simulink subsystem "subsys_Full_Model_NL"  (R2021a)
settings: Solver=VariableStepAuto  StartTime=0.0  StopTime=10.0  RelTol=1e-3
values from neighbouring files (symbols this model uses):
  g = 9.81    [Constante_NL.m]
  LL = .115    (= 0.115)    [Constante_NL.m]
  mP = masseP    (= 0.425)    [Constante_NL.m]
  RR = 3.6    [Constante_NL.m]
  sig = 1    [Constante_NL.m]
  XA = +rABC    (= 0.0952)    [Constante_NL.m]
  XB = -rABC*sind(30)    [Constante_NL.m]
  XC = -rABC*sind(30)    [Constante_NL.m]
  XD = +rDEF*sind(30)    [Constante_NL.m]
  XE = -rDEF    (= -0.08)    [Constante_NL.m]
  XF = +rDEF*sind(30)    [Constante_NL.m]
  YA = 0.0    (= 0)    [Constante_NL.m]
  YB = +rABC*cosd(30)    [Constante_NL.m]
  YC = -rABC*cosd(30)    [Constante_NL.m]
  YD = +rDEF*cosd(30)    [Constante_NL.m]
  YE = 0.0    (= 0)    [Constante_NL.m]
  YF = -rDEF*cosd(30)    [Constante_NL.m]
undefined symbols (not defined in the file or in its folder): Jx, mS
settings Model: Creator=antho  LastModifiedBy=antho

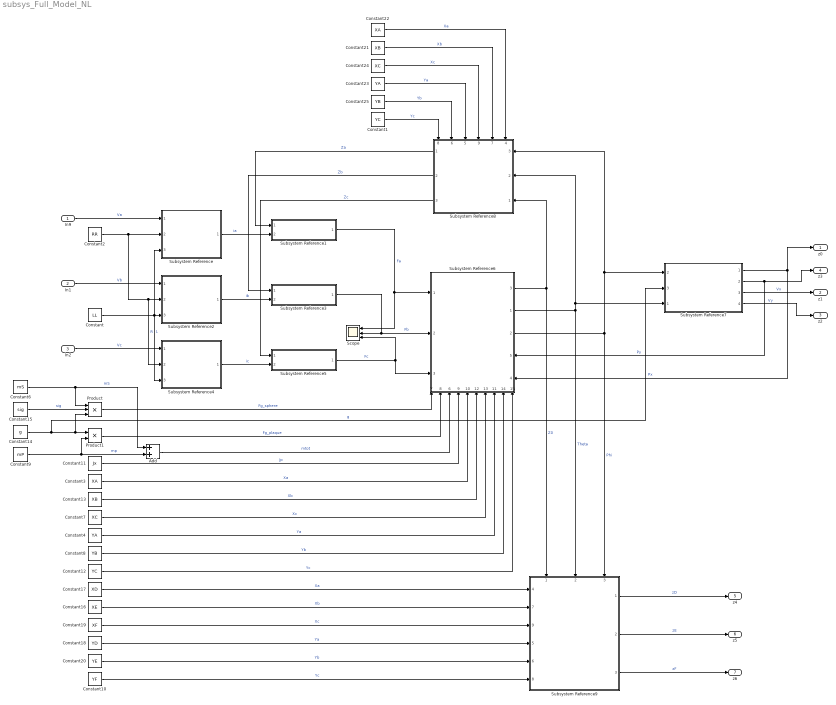
== system subsys_Full_Model_NL ==
  In9 : Inport
  In1 : Inport  Port=2
  In2 : Inport  Port=3
  Add : Sum
  Constant : Constant  Value=LL
  Constant1 : Constant  Value=YC
  Constant10 : Constant  Value=YF
  Constant11 : Constant  Value=Jx
  Constant12 : Constant  Value=YC
  Constant13 : Constant  Value=XB
  Constant14 : Constant  Value=g
  Constant15 : Constant  Value=sig
  Constant16 : Constant  Value=XE
  Constant17 : Constant  Value=XD
  Constant18 : Constant  Value=YD
  Constant19 : Constant  Value=XF
  Constant2 : Constant  Value=RR
  Constant20 : Constant  Value=YE
  Constant21 : Constant  Value=XB
  Constant22 : Constant  Value=XA
  Constant23 : Constant  Value=YA
  Constant24 : Constant  Value=XC
  Constant25 : Constant  Value=YB
  Constant3 : Constant  Value=XA
  Constant4 : Constant  Value=YA
  Constant6 : Constant  Value=mS
  Constant7 : Constant  Value=XC
  Constant8 : Constant  Value=YB
  Constant9 : Constant  Value=mP
  Product : Product  Inputs=3
  Product1 : Product
  Scope : Scope  NumInputPorts=3
  Subsystem Reference : Subsystem  ReferencedSubsystem=subsys_courant
  Subsystem Reference1 : Subsystem  ReferencedSubsystem=subsys_force_2
  Subsystem Reference2 : Subsystem  ReferencedSubsystem=subsys_courant
  Subsystem Reference3 : Subsystem  ReferencedSubsystem=subsys_force_2
  Subsystem Reference4 : Subsystem  ReferencedSubsystem=subsys_courant
  Subsystem Reference5 : Subsystem  ReferencedSubsystem=subsys_force_2
  Subsystem Reference6 : Subsystem  ReferencedSubsystem=subsys_dynamic_plaque
      settings: PortSchema="{\"entries\":[{\"content\":{\"sides\":[{\"content\":{\"connectorIds\":[\"In1\",\"In2\",\"In3\"]},\"type\":\"ConnectorPlacement.EquallySpacedRectSide\",\"uuid\":\"ca40e79e-dd52-4e81-b398-9363b7d09f0b\"},{\"content\":{\"connectorIds\":[\"Out3\",\"Out1\",\"Out2\",\"In5\",\"In4\"],\"side\":\"RIGHT\"},\"type\":\"ConnectorPlacement.EquallySpacedRectSide\",\"uuid\":\"1099d2b9-47c5-4719-b254-466629c51b1a\"},{\"content\":{\"connectorIds\":[],\"side\":\"TOP\"},\"type\":\"ConnectorPlacement.EquallySpacedRectSide\",\"uuid\":\"da25c805-e43e-4efa-b3d1-32b5e54c3b7e\"},{\"content\":{\"connectorIds\":[\"In7\",\"In8\",\"In6\",\"In9\",\"In10\",\"In12\",\"In13\",\"In11\",\"In14\",\"In15\"],\"side\":\"BOTTOM\"},\"type\":\"ConnectorPlacement.EquallySpacedRectSide\",\"uuid\":\"c9de39aa-1a48-4d35-8587-898aa5305618\"}]},\"type\":\"ConnectorPlacement.EquallySpacedConnector\",\"uuid\":\"5a66023b-e172-4aa2-bb07-18c38d101412\"}],\"packageUris\":[\"http://schema.mathworks.com/mf0/Connector/R2020b\"],\"version\":\"1.0\"}"
  Subsystem Reference7 : Subsystem  ReferencedSubsystem=subsys_sphere_position
      settings: PortSchema="{\"entries\":[{\"content\":{\"sides\":[{\"content\":{\"connectorIds\":[\"In2\",\"In3\",\"In1\"]},\"type\":\"ConnectorPlacement.EquallySpacedRectSide\",\"uuid\":\"96a04a08-4352-43c8-a8bd-dce0633e76dd\"},{\"content\":{\"connectorIds\":[\"Out1\",\"Out2\",\"Out3\",\"Out4\"],\"side\":\"RIGHT\"},\"type\":\"ConnectorPlacement.EquallySpacedRectSide\",\"uuid\":\"6371aec0-efd7-4766-a972-236c23c9f028\"},{\"content\":{\"connectorIds\":[],\"side\":\"TOP\"},\"type\":\"ConnectorPlacement.EquallySpacedRectSide\",\"uuid\":\"d707f900-e5a5-42aa-a3e1-854061b3e5bc\"}]},\"type\":\"ConnectorPlacement.EquallySpacedConnector\",\"uuid\":\"29279e07-6ad8-4183-91e5-486e6736f1f9\"}],\"packageUris\":[\"http://schema.mathworks.com/mf0/Connector/R2020b\"],\"version\":\"1.0\"}"
  Subsystem Reference8 : Subsystem  ReferencedSubsystem=Hauteur_Aimants_Plaque_2
      settings: PortSchema="{\"entries\":[{\"content\":{\"sides\":[{\"content\":{\"connectorIds\":[\"In3\",\"In2\",\"In1\"]},\"type\":\"ConnectorPlacement.EquallySpacedRectSide\",\"uuid\":\"aad0297c-2a16-40e4-ae4d-ded4810484bd\"},{\"content\":{\"connectorIds\":[\"Out1\",\"Out2\",\"Out3\"],\"side\":\"RIGHT\"},\"type\":\"ConnectorPlacement.EquallySpacedRectSide\",\"uuid\":\"a548181b-8d4f-4e8c-8e81-e157a1504375\"},{\"content\":{\"connectorIds\":[\"In4\",\"In7\",\"In9\",\"In5\",\"In6\",\"In8\"],\"side\":\"TOP\"},\"type\":\"ConnectorPlacement.EquallySpacedRectSide\",\"uuid\":\"36d9bd6e-86ec-486f-98ec-c4e19d794fba\"}]},\"type\":\"ConnectorPlacement.EquallySpacedConnector\",\"uuid\":\"cbff7459-b836-4b55-8a47-eadd2f910e6f\"}],\"packageUris\":[\"http://schema.mathworks.com/mf0/Connector/R2020b\"],\"version\":\"1.0\"}"
  Subsystem Reference9 : Subsystem  ReferencedSubsystem=subsys_calcul_capteurs
      settings: PortSchema="{\"entries\":[{\"content\":{\"sides\":[{\"content\":{\"connectorIds\":[\"In4\",\"In7\",\"In9\",\"In5\",\"In6\",\"In8\"]},\"type\":\"ConnectorPlacement.EquallySpacedRectSide\",\"uuid\":\"47cb094f-47d2-4ed2-aeac-cf8db82fb2e1\"},{\"content\":{\"connectorIds\":[\"Out1\",\"Out2\",\"Out3\"],\"side\":\"RIGHT\"},\"type\":\"ConnectorPlacement.EquallySpacedRectSide\",\"uuid\":\"0d967583-d7cd-45d7-99e9-aa009bb95853\"},{\"content\":{\"connectorIds\":[\"In1\",\"In2\",\"In3\"],\"side\":\"TOP\"},\"type\":\"ConnectorPlacement.EquallySpacedRectSide\",\"uuid\":\"443c4f5e-938a-4a87-b4d7-addf09620ce5\"}]},\"type\":\"ConnectorPlacement.EquallySpacedConnector\",\"uuid\":\"baf65586-56dd-438f-8f73-6675f8191181\"}],\"packageUris\":[\"http://schema.mathworks.com/mf0/Connector/R2020b\"],\"version\":\"1.0\"}"
  z0 : Outport
  z1 : Outport  Port=2
  z2 : Outport  Port=3
  z3 : Outport  Port=4
  z4 : Outport  Port=5
  z5 : Outport  Port=6
  z6 : Outport  Port=7
  wires:
  Subsystem Reference8/2 -> Subsystem Reference3/1  "Zb"
  Subsystem Reference7/1 -> Subsystem Reference6/4, z0/1  "Px"
  Constant7/1 -> Subsystem Reference6/13  "Xc"
  Constant4/1 -> Subsystem Reference6/11  "Ya"
  In2/1 -> Subsystem Reference4/1  "Vc"
  Subsystem Reference5/1 -> Scope/3, Subsystem Reference6/3  "Fc"
  Subsystem Reference/1 -> Subsystem Reference1/2  "ia"
  Constant8/1 -> Subsystem Reference6/14  "Yb"
  In1/1 -> Subsystem Reference2/1  "Vb"
  Subsystem Reference6/3 -> Subsystem Reference8/1, Subsystem Reference9/1  "Z0"
  Constant9/1 -> Product1/2, Add/2  "mp"
  Subsystem Reference2/1 -> Subsystem Reference3/2  "ib"
  Product/1 -> Subsystem Reference6/7  "Fg_sphere"
  Constant3/1 -> Subsystem Reference6/10  "Xa"
  Subsystem Reference7/2 -> z3/1, Subsystem Reference6/5  "Py"
  Subsystem Reference8/1 -> Subsystem Reference1/1  "Za"
  Constant12/1 -> Subsystem Reference6/15  "Yc"
  Constant11/1 -> Subsystem Reference6/9  "Jp"
  Constant2/1 -> Subsystem Reference/2, Subsystem Reference2/2, Subsystem Reference4/2  "R"
  Subsystem Reference7/4 -> z2/1  "Vy"
  Subsystem Reference6/1 -> Subsystem Reference7/1, Subsystem Reference8/2, Subsystem Reference9/2  "Theta"
  Subsystem Reference4/1 -> Subsystem Reference5/2  "ic"
  Subsystem Reference3/1 -> Scope/2, Subsystem Reference6/2  "Fb"
  Subsystem Reference8/3 -> Subsystem Reference5/1  "Zc"
  Subsystem Reference6/2 -> Subsystem Reference9/3, Subsystem Reference7/2, Subsystem Reference8/3  "Phi"
  In9/1 -> Subsystem Reference/1  "Va"
  Constant/1 -> Subsystem Reference/3, Subsystem Reference4/3, Subsystem Reference2/3  "L"
  Subsystem Reference1/1 -> Scope/1, Subsystem Reference6/1  "Fa"
  Product1/1 -> Subsystem Reference6/8  "Fg_plaque"
  Constant13/1 -> Subsystem Reference6/12  "Xb"
  Subsystem Reference7/3 -> z1/1  "Vx"
  Constant14/1 -> Product1/1, Product/3, Subsystem Reference7/3  "g"
  Constant6/1 -> Add/1, Product/1  "mS"
  Constant15/1 -> Product/2  "sig"
  Constant17/1 -> Subsystem Reference9/4  "Xa"
  Subsystem Reference9/1 -> z4/1  "zD"
  Subsystem Reference9/2 -> z5/1  "zE"
  Subsystem Reference9/3 -> z6/1  "zF"
  Add/1 -> Subsystem Reference6/6  "mtot"
  Constant16/1 -> Subsystem Reference9/7  "Xb"
  Constant19/1 -> Subsystem Reference9/9  "Xc"
  Constant18/1 -> Subsystem Reference9/5  "Ya"
  Constant20/1 -> Subsystem Reference9/6  "Yb"
  Constant10/1 -> Subsystem Reference9/8  "Yc"
  Constant22/1 -> Subsystem Reference8/4  "Xa"
  Constant21/1 -> Subsystem Reference8/7  "Xb"
  Constant24/1 -> Subsystem Reference8/9  "Xc"
  Constant23/1 -> Subsystem Reference8/5  "Ya"
  Constant25/1 -> Subsystem Reference8/6  "Yb"
  Constant1/1 -> Subsystem Reference8/8  "Yc"
